simulink model "nonlinearstm"  (R2018b)
settings: configuration reference "Physics" (kept outside this file)
model workspace (MAT data in the model file):
  veh_param = Simulink.Parameter
  veh_param.Value.cLiftF = 0
  veh_param.Value.cLiftR = 0
  veh_param.Value.CoGx_m = 0
  veh_param.Value.CoGy_m = 0
  veh_param.Value.CoGz_m = 0
  veh_param.Value.cDrag = 0
  veh_param.Value.Aref_m2 = 0
  veh_param.Value.Gearratio = 0
  veh_param.Value.Wheelbase_m = 0
  veh_param.Value.PacLatF = [0 0 0 0 0]
  veh_param.Value.PacLongF = [0 0 0 0 0]
  veh_param.Value.PacLatR = [0 0 0 0 0]
  veh_param.Value.PacLongR = [0 0 0 0 0]
  veh_param.Value.cRollFriction_Npmps = 0
  veh_param.Value.MaxRollFriction_N = 0
  veh_param.Value.T_YawRate_s = 0
  veh_param.Value.T_LatVel_s = 0
  veh_param.Value.TrackWidthF_m = 0
  veh_param.Value.TrackWidthR_m = 0
  veh_param.Value.TireRadiusF_m = 0
  veh_param.Value.TireRadiusR_m = 0
  veh_param.Value.VehicleInertia_kgm2 = 0
  veh_param.Value.WheelInertiaF_kgm2 = 0
  veh_param.Value.WheelInertiaR_kgm2 = 0
  veh_param.Value.VehicleMass_kg = 0
  veh_param.Value.switchModelBlend_mps = 0
  veh_param.Value.PTLimitLowVel_N = 0
  veh_param.Value.switchModelVel_mps = 0
  veh_param.Value.T_Tire_s = 0
  veh_param.DataType = 'struct'
  veh_param.Dimensions = [1 1]
  x0_positionstates = Simulink.Parameter
  x0_positionstates.Value = [0 0 0]
  x0_positionstates.DataType = 'auto'
  x0_positionstates.Dimensions = [1 3]
undefined symbols (not defined in the file): x0_vehiclestates
settings Model: DataDictionary=nonlinearstm.sldd  ParameterArgumentNames=veh_param,x0_positionstates  Creator=wischnewski  LastModifiedBy=ge34qer

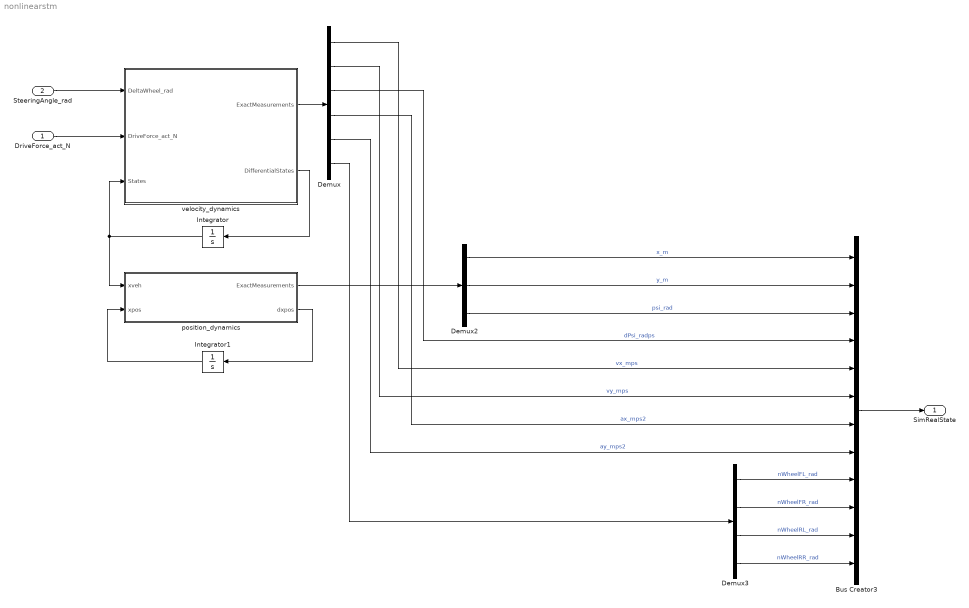
== system nonlinearstm ==
  DriveForce_act_N : Inport  OutDataTypeStr=Bus: DriveForce_N
  SteeringAngle_rad : Inport  Port=2
  Bus Creator3 : BusCreator  Inputs=12  OutDataTypeStr=Bus: SimRealState
  Demux : Demux  Outputs=[1 1 1 1 1 4]
  Demux2 : Demux  Outputs=3
  Demux3 : Demux
  Integrator : Integrator  InitialCondition=x0_vehiclestates
  Integrator1 : Integrator  InitialCondition=x0_positionstates
  position_dynamics : MATLAB Function  TreatAsAtomicUnit=on
  velocity_dynamics : MATLAB Function  TreatAsAtomicUnit=on
  SimRealState : Outport  OutDataTypeStr=Bus: SimRealState
  wires:
  Demux/1 -> Bus Creator3/5  "vx_mps"
  Integrator1/1 -> position_dynamics/2(xpos)
  position_dynamics/2(dxpos) -> Integrator1/1
  position_dynamics/1(ExactMeasurements) -> Demux2/1
  Demux/2 -> Bus Creator3/6  "vy_mps"
  Demux2/3 -> Bus Creator3/3  "psi_rad"
  Demux/3 -> Bus Creator3/4  "dPsi_radps"
  Demux/4 -> Bus Creator3/7  "ax_mps2"
  Demux/5 -> Bus Creator3/8  "ay_mps2"
  Demux2/1 -> Bus Creator3/1  "x_m"
  Demux2/2 -> Bus Creator3/2  "y_m"
  velocity_dynamics/1(ExactMeasurements) -> Demux/1
  velocity_dynamics/2(DifferentialStates) -> Integrator/1
  Integrator/1 -> velocity_dynamics/3(States), position_dynamics/1(xveh)
  SteeringAngle_rad/1 -> velocity_dynamics/1(DeltaWheel_rad)
  Demux/6 -> Demux3/1
  DriveForce_act_N/1 -> velocity_dynamics/2(DriveForce_act_N)
  Bus Creator3/1 -> SimRealState/1
  Demux3/1 -> Bus Creator3/9  "nWheelFL_rad"
  Demux3/2 -> Bus Creator3/10  "nWheelFR_rad"
  Demux3/4 -> Bus Creator3/12  "nWheelRR_rad"
  Demux3/3 -> Bus Creator3/11  "nWheelRL_rad"

== matlab function nonlinearstm/velocity_dynamics ==
  data: ExactMeasurements output; DeltaWheel_rad input; DriveForce_act_N input Bus: DriveForce_N; DifferentialStates output; States input; veh_param parameter Bus: VehicleParameterSet
function [ExactMeasurements, DifferentialStates] = fcn(DeltaWheel_rad, DriveForce_act_N, States, veh_param)

[ExactMeasurements, DifferentialStates] = VehicleModel(DeltaWheel_rad, DriveForce_act_N, States, veh_param);

== matlab function nonlinearstm/position_dynamics ==
  data: ExactMeasurements output; xveh input; xpos input; dxpos output
function [ExactMeasurements, dxpos] = fcn(xveh, xpos)

[ExactMeasurements, dxpos] = PositionModel(xveh, xpos);
